simulink model "color_acquistion_test"  (R2022b)
settings: Solver=FixedStepDiscrete  StartTime=0.0  StopTime=10000.0  FixedStep=0.1  RelTol=1e-3
InitFcn:
  | mbd_s32k_consistency_checks(bdroot(gcs));
undefined symbols (not defined in the file or in its folder): LQFP
libraries: mbd_s32k1xx_ec_toolbox x5
settings Model: Creator=leona  LastModifiedBy=leona
settings DataIOCC: SaveOutput=off  SignalLogging=off  SaveTime=off
settings OptimizationCC: DefaultParameterBehavior=Inlined  EnhancedBackFolding=on  PassReuseOutputArgsAs=Individual arguments  ZeroExternalMemoryAtStartup=off  ZeroInternalMemoryAtStartup=off  OptimizeBlockOrder=speed  DifferentSizesBufferReuse=on  OptimizationCustomize=off  EfficientTunableParamExpr=on
settings DebuggingCC: InheritedTsInSrcMsg=none  SingleTaskRateTransMsg=error  ParameterTunabilityLossMsg=error  UnconnectedInputMsg=error  UnconnectedOutputMsg=error  UnconnectedLineMsg=error  UnknownTsInhSupMsg=error
settings HardwareCC: ProdBitPerPointer=32  ProdBitPerSizeT=32  ProdBitPerPtrDiffT=32  ProdLargestAtomicInteger=Long  ProdLargestAtomicFloat=Double  ProdWordSize=32  ProdHWDeviceType=ARM Compatible->ARM Cortex
settings ModelReferenceCC: ModelReferenceNumInstancesAllowed=Single
settings SFSimCC: MATLABDynamicMemAlloc=off
settings RTWCC: Description=Model Based Design Toolbox S32K1xx Code Generation Target  SystemTargetFile=mbd_s32k.tlc  MakeCommand=mbd_s32k_make_rtw COPY_MDLREF_INCLUDES=0  TemplateMakefile=mbd_s32k.tmf
settings CodeAppCC: ForceParamTrailComments=on  IgnoreCustomStorageClasses=off  OperatorAnnotations=on  SimulinkDataObjDesc=on  SFDataObjDesc=on  InsertBlockDesc=on
settings STFCustomTargetCC: TargetLangStandard=C99 (ISO)  MultiwordLength=256  CombineOutputUpdateFcns=on  ERTCustomFileBanners=on  SupportContinuousTime=off  SupportNonInlinedSFcns=off  RemoveResetFunc=on  MATLABClassNameForMDSCustomization=Simulink.SoftwareTarget.ERTCustomization  SystemTargetFile=mbd_s32k.tlc
settings ERTTargetCC: TargetLangStandard=C99 (ISO)  ParMdlRefBuildCompliant=off  CompOptLevelCompliant=off  ConcurrentExecutionCompliant=off  ModelStepFunctionPrototypeControlCompliant=off  CPPClassGenCompliant=off  UseToolchainInfoCompliant=off  ExtMode=on  InlinedParameterPlacement=NonHierarchical  ERTSrcFileBannerTemplate=mbd_ert_code_template.cgt  ERTHdrFileBannerTemplate=mbd_ert_code_template.cgt  ERTDataSrcFileTemplate=mbd_ert_code_template.cgt  ERTDataHdrFileTemplate=mbd_ert_code_template.cgt  ERTCustomFileTemplate=example_file_process.tlc

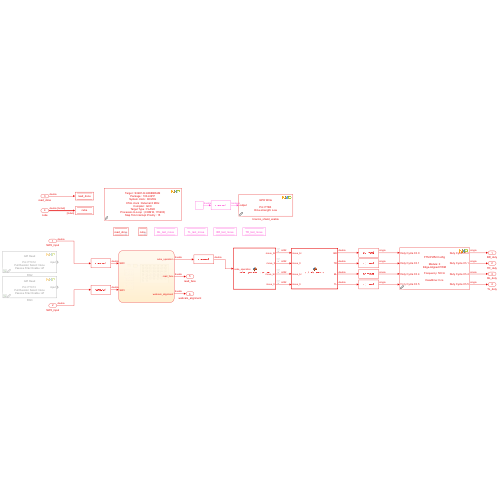
[thumbnail: Simulink's stored preview of the top-level diagram]
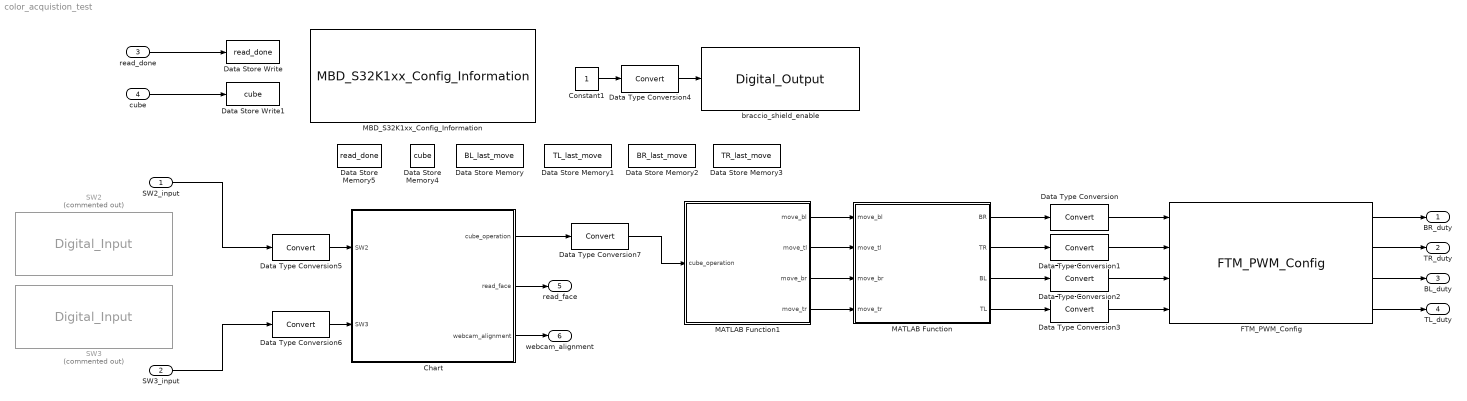
== system color_acquistion_test ==
  SW2_input : Inport
  SW3_input : Inport  Port=2
  read_done : Inport  Port=3
  cube : Inport  Port=4
  Chart : Stateflow chart  TreatAsAtomicUnit=on
  Constant1 : Constant
  Data Store Memory : DataStoreMemory  DataStoreName=BL_last_move  WriteAfterWriteMsg=warning  ShowAdditionalParam=off
  Data Store Memory1 : DataStoreMemory  DataStoreName=TL_last_move  WriteAfterWriteMsg=warning  ShowAdditionalParam=off
  Data Store Memory2 : DataStoreMemory  DataStoreName=BR_last_move  WriteAfterWriteMsg=warning  ShowAdditionalParam=off
  Data Store Memory3 : DataStoreMemory  DataStoreName=TR_last_move  WriteAfterWriteMsg=warning  ShowAdditionalParam=off
  Data Store Memory4 : DataStoreMemory  DataStoreName=cube  WriteAfterWriteMsg=warning  InitialValue=zeros(3, 3, 6)  VectorParams1D=off  ShowAdditionalParam=off  OutDataTypeStr=double
  Data Store Memory5 : DataStoreMemory  DataStoreName=read_done  WriteAfterWriteMsg=warning  ShowAdditionalParam=off  OutDataTypeStr=double
  Data Store Write : DataStoreWrite  DataStoreName=read_done  IndexOptions=Index vector (dialog)  Indices=1  OutputSizes=1
  Data Store Write1 : DataStoreWrite  DataStoreName=cube  IndexOptions=Index vector (dialog)  Indices=1  OutputSizes=1
  Data Type Conversion{,1..7} (8 alike) : DataTypeConversion  SaturateOnIntegerOverflow=off  RndMeth=Floor
  FTM_PWM_Config : mbd_s32k1xx_ec_toolbox/Motor Control Blocks/FTM Blocks/FTM_PWM_Config  ftmModule=0  ftmMode=Edge-Aligned PWM  ftmSourceClock=80 MHz  swcontrol_enable=off  chan0En=on  chan0Type=Independent  chan2En=off  chan2Type=Independent  chan4En=on  chan4Type=Independent  chan6En=off  chan6Type=Independent  ftmPwmUnits=Hz  outFrequency=50  ftmPeriod=25000  ftmPrescaler=Divide by 64  deadtimeUnits=Nanoseconds  deadtimeNs=0  deadtimeTicks=0  deadtimePrescaler=Divide by 1  dutyCycleCh0=0.03  dutyCycleCh1=0.125  dutyCycleCh2=0.025  dutyCycleCh3=0.025  dutyCycleCh4=0.025  dutyCycleCh5=0.025  dutyCycleCh6=0.25  dutyCycleCh7=0.25  dutyCycleSim=on  startAfterInit=on  showAdvOpt=on  pinFtmCh0=PTD15: [FTM0_CH0 | FTM Channel]  pinFtmCh1=PTD16: [FTM0_CH1 | FTM Channel]  pinPolCh0=Active High  pinPolCh1=Active High  outputComplem0=Main duplicated  outputLevel0=Low  outputLevel1=Low  pinFtmCh2=PTB14: [FTM0_CH2 | FTM Channel]  pinFtmCh3=PTC3: [FTM0_CH3 | FTM Channel]  pinPolCh2=Active High  pinPolCh3=Active High  outputComplem2=Main duplicated  outputLevel2=Low  outputLevel3=Low  pinFtmCh4=PTB4: [FTM0_CH4 | FTM Channel]  pinFtmCh5=PTB5: [FTM0_CH5 | FTM Channel]  pinPolCh4=Active High  pinPolCh5=Active High  outputComplem4=Main duplicated  outputLevel4=Low  outputLevel5=Low  pinFtmCh6=PTE8: [FTM0_CH6 | FTM Channel]  pinFtmCh7=None  pinPolCh6=Active High  pinPolCh7=Active High  outputComplem6=Main duplicated  outputLevel6=Low  outputLevel7=Low  initTrigger=off  chTrigger0=off  chTrigger1=off  chTrigger2=off  chTrigger3=off  chTrigger4=off  chTrigger5=off  chTrigger6=off  chTrigger7=off  mcuTargetUpdate=on  pwmSyncTrg=Software trigger  pwmSyncHwRouting=TRGMUX_FTM7  pwmSyncTrg0=off  pwmSyncTrg1=off  pwmSyncTrg2=off  pwmSyncAutoClear=on  pwmSyncMinLoad=on  pwmSyncMaxLoad=on  pwmSyncInvert=System Clock  pwmSyncOutControl=System Clock  pwmSyncOutMask=System Clock  pwmSyncCounterInitial=System Clock  pwmSyncPoints=Update now  reloadEnable=off  reloadPriority=15  reloadHalfCycle=off  reloadHCR=0  reloadFrequency=0  chnMatch0=off  chnMatch1=off  chnMatch2=off  chnMatch3=off  chnMatch4=off  chnMatch5=off  chnMatch6=off  chnMatch7=off  pwmFaultProtection=off  pwmFaultInterrupt=off  pwmFaultClearing=Fault control disabled  pwmFaultPinState=Safe Value  pwmFaultFilterValue=0  pwmFaultPriority=15  fault_disen_0=off  fault_filter_0=off  fault_polarity_0=Active High  fault_disen_1=off  fault_filter_1=off  fault_polarity_1=Active high  fault_disen_2=off  fault_filter_2=off  fault_polarity_2=Active high  fault_disen_3=off  fault_filter_3=off  fault_polarity_3=Active high  fault_pin_0=None  fault_pin_1=None  fault_pin_2=None  fault_pin_3=None
  MATLAB Function : MATLAB Function  TreatAsAtomicUnit=on
  MATLAB Function1 : MATLAB Function  TreatAsAtomicUnit=on
  MBD_S32K1xx_Config_Information : mbd_s32k1xx_ec_toolbox/MBD_S32K1xx_Config_Information  mbdt_ver=0  disp_str=|  config_params=[]  mcu_target_name=S32K144  mcu_target_package=100-LQFP  mcu_target_sram_size=48KB  mcu_system_clock_freq=80  mcu_xtal_freq=External 8  mcu_steptick_timer=LPIT Channel 0  mcu_steptick_prio=15  ds_import_enable=on  target_compiler=GCC  target_memory=FLASH  gcc_target_compile_opts=-mthumb -mfloat-abi=hard -mfpu=fpv4-sp-d16 -O1 -g -gstrict-dwarf  gcc_target_assemble_opts=-mthumb -mfloat-abi=hard -mfpu=fpv4-sp-d16 -g  gcc_target_link_opts=-mthumb -mfloat-abi=hard -mfpu=fpv4-sp-d16  gcc_target_default_lcf=on  gcc_target_user_lcf=S32K144_48_flash.ld  ghs_target_compile_opts=-cpu=cortexm4f -thumb -fpu=vfpv4_d16 -fsingle -Ogeneral -Wundef -Wimplicit-int -Wshadow -Wtrigraphs --no_commons --gnu_asm -gnu99 -gdwarf-2 -G  ghs_target_assemble_opts=-cpu=cortexm4f -fpu=vfpv4_d16  ghs_target_link_opts=-cpu=cortexm4f -thumb -fpu=vfpv4_d16  ghs_target_default_lcf=on  ghs_target_user_lcf=S32K144_48_flash.ld  iar_target_compile_opts=--cpu=Cortex-M4F --thumb --fpu=VFPv4_sp -Ol -e --debug --dlib_config normal  iar_target_assemble_opts=--cpu Cortex-M4F --thumb --fpu VFPv4_sp  iar_target_link_opts=--no_exceptions --vfe --inline  iar_target_default_lcf=on  iar_target_user_lcf=S32K144_48_flash.icf  pil_download_enable=on  rbl_download_enable=on  rbl_start_delay=5000  rbl_download_interface=OpenSDA  rbl_restart_request=off  rbl_com_port=Custom  rbl_com_port_custom=COM18  pil_download_rate=115200  pil_download_rate_custom=115200  pil_opensda_drive=Custom  pil_opensda_drive_custom=D  jtag_interface=OpenSDA Embedded Debug  jlink_default_path=on  jlink_user_path=C:\Program Files\SEGGER\JLink\  pil_uart_instance=1  pil_uart_rx=PTC6: [LPUART1_RX | Receive]  pil_uart_tx=PTC7: [LPUART1_TX | Transmit]  FTM_PWM_PcrCheckEnDis=on  FTM_Input_Edge_Inputs_PcrCheckEnDis=on  FTM_Dual_Edge_Inputs_PcrCheckEnDis=on  FTM_Quadrature_Inputs_PcrCheckEnDis=on  FTM_Hall_Sensor_Inputs_PcrCheckEnDis=on  LPTMR_PcrCheckEnDis=on  PIT_PcrCheckEnDis=on  RTC_PcrCheckEnDis=on  FlexCAN_PcrCheckEnDis=on  LIN_PcrCheckEnDis=on  FlexIO_PcrCheckEnDis=on  LPI2C_PcrCheckEnDis=on  LPSPI_PcrCheckEnDis=on  LPUART_PcrCheckEnDis=on  CMP_PcrCheckEnDis=on  GPIO_OutputPcrCheckEnDis=on  GPIO_InputPcrCheckEnDis=on  SBC_PcrCheckEnDis=on  BMS_PcrCheckEnDis=on  AMMCLIB_PcrCheckEnDis=on  FM_PcrCheckEnDis=on  Profile_PcrCheckEnDis=on  ConfigParams_PcrCheckEnDis=on  ModelRef_PcrCheckEnDis=on  PDB0_PcrCheckEnDis=on  CSEc_PcrCheckEnDis=on  eDMA_PcrCheckEnDis=on  FLASH_PcrCheckEnDis=on  ADC_PcrCheckEnDis=on  WDOG_PcrCheckEnDis=on
      | Target : S32K144-64KB_SRAM
      | Package : 100-pin
      | System clock : 80 MHz
      | XTAL clock : External 8 MHz
      | Compiler : IAR
      | Target Type : FLASH
      | Download Code after build : off
      | Step Tick Interrupt Priority : 15
  SW2 : mbd_s32k1xx_ec_toolbox/GPIO Blocks/Digital_Input  Commented=on  gpio_pin=PTC12: [PTC12 | Port C I/O]  pull_resistor=None  passive_filter=off
  SW3 : mbd_s32k1xx_ec_toolbox/GPIO Blocks/Digital_Input  Commented=on  gpio_pin=PTC13: [PTC13 | Port C I/O]  pull_resistor=None  passive_filter=off
  braccio_shield_enable : mbd_s32k1xx_ec_toolbox/GPIO Blocks/Digital_Output  gpio_pin=PTB3: [PTB3 | Port B I/O]  init_val=Low  drive_strength=Low
  BR_duty : Outport
  TR_duty : Outport  Port=2
  BL_duty : Outport  Port=3
  TL_duty : Outport  Port=4
  read_face : Outport  Port=5
  webcam_alignment : Outport  Port=6
  wires:
  Data Type Conversion2/1 -> FTM_PWM_Config/3
  MATLAB Function1/3(move_br) -> MATLAB Function/3(move_br)
  FTM_PWM_Config/1 -> BR_duty/1
  MATLAB Function/4(TL) -> Data Type Conversion3/1
  FTM_PWM_Config/2 -> TR_duty/1
  Data Type Conversion5/1 -> Chart/1(SW2)
  Data Type Conversion4/1 -> braccio_shield_enable/1
  MATLAB Function/3(BL) -> Data Type Conversion2/1
  Chart/1(cube_operation) -> Data Type Conversion7/1
  Constant1/1 -> Data Type Conversion4/1
  MATLAB Function/1(BR) -> Data Type Conversion/1
  MATLAB Function1/1(move_bl) -> MATLAB Function/1(move_bl)
  FTM_PWM_Config/4 -> TL_duty/1
  Data Type Conversion7/1 -> MATLAB Function1/1(cube_operation)
  FTM_PWM_Config/3 -> BL_duty/1
  Data Type Conversion3/1 -> FTM_PWM_Config/4
  MATLAB Function/2(TR) -> Data Type Conversion1/1
  Data Type Conversion6/1 -> Chart/2(SW3)
  Data Type Conversion1/1 -> FTM_PWM_Config/2
  MATLAB Function1/4(move_tr) -> MATLAB Function/4(move_tr)
  Data Type Conversion/1 -> FTM_PWM_Config/1
  MATLAB Function1/2(move_tl) -> MATLAB Function/2(move_tl)
  SW2_input/1 -> Data Type Conversion5/1
  SW3_input/1 -> Data Type Conversion6/1
  Chart/2(read_face) -> read_face/1
  Chart/3(webcam_alignment) -> webcam_alignment/1
  read_done/1 -> Data Store Write/1
  cube/1 -> Data Store Write1/1

== matlab function color_acquistion_test/MATLAB Function1 ==
  data: cube_operation input; move_bl output; move_tl output; move_br output; move_tr output
function [move_bl, move_tl, move_br, move_tr] = cube_operation_decoder(cube_operation)
% This function takes as input the code for a cube operation and converts
% it as positions of the 4 servo motors. The operations must be a 4 digit
% unsigned integer, encoded as follows:
%   - first digit [0, 1]: open/close left grip;
%   - second digit [0, 1]: open/close right grip;
%   - third digit [0, 1, 2]: set left arm to 90/0/180 degrees
%   - fourth digit [0, 1, 2]: set right arm to 90/0/180 degress

x1 = int32(mod(cube_operation/1000, 10));
x2 = int32(mod(cube_operation/100, 10));
x3 = int32(mod(cube_operation/10, 10));
x4 = int32(mod(cube_operation, 10));

move_tl = x1;
move_tr = x2;
move_bl = x3;
move_br = x4;

== matlab function color_acquistion_test/MATLAB Function ==
  data: BR output; TR output; move_bl input; BL output; move_tl input; move_br input; move_tr input; TL output
function [BR, TR, BL, TL] = actuate_servos(move_bl, move_tl, move_br, move_tr)
% This function takes as input as specific number associated to a movement
% of the 4 servo motors (BL = Bottom Left, TL = Top Left, BR = Bottom Right,
% TR = Top Right) and it gives as output the 4 relative duty cycles needed to
% obtain that movement. 

min_duty = 0.025;
max_duty = 0.125;

duty_0_deg = min_duty;
duty_grip_open = min_duty + (max_duty-min_duty)/3;
duty_grip_closed = min_duty + (max_duty-min_duty)/15; 
duty_90_deg = min_duty + (max_duty-min_duty)/2;
duty_180_deg = max_duty;

switch (move_tl)
    case 0                  % Open left grip
        TL = duty_grip_open;
    case 1                  % Close left grip
        TL = duty_grip_closed;
    otherwise               % Open left grip
        TL = duty_grip_open;
end

switch (move_tr)
    case 0                  % Open right grip
        TR = duty_grip_open;
    case 1                  % Close right grip
        TR = duty_grip_closed;
    otherwise               % Open right grip
        TR = duty_grip_open;
end

switch (move_bl)
    case 0                  % Left arm straight
        BL = duty_90_deg;
    case 1                  % Left arm at 90° clockwise
        BL = duty_0_deg;
    case 2                 % Left arm at 90° counter-clockwise
        BL = duty_180_deg;
    otherwise
        BL = duty_90_deg;
end

switch (move_br)
    case 0                  % Right arm straight
        BR = duty_90_deg;
    case 1                  % Right arm at 90° clockwise
        BR = duty_0_deg;
    case 2                 % Right arm at 90° counter-clockwise
        BR = duty_180_deg;
    otherwise
        BR = duty_90_deg;
end

% Update current position of the motors
BL_last_move = move_bl;
TL_last_move = move_tl;
BR_last_move = move_br;
TR_last_move = move_tr;

== stateflow chart color_acquistion_test/Chart ==
  state read_cube
    en:
    webcam_alignment = 0;
    % Clear cube colors
    cube = zeros(3, 3, 6);
    %read red
    %LTm
    %read blue
    %LTm
    %read orange
    %LTm
    %read green
    %RTm
    %LTm
    %read white
    %RTmm
    %LTmm
    %read yellow
    %RTm
    %LTm
    %RTp
    state read_red
      en:
    state fase1e
      en:
      cube_operation=1000
    state fase2e
      en:
      cube_operation=1010
    state fase3e
      en:
      cube_operation=1110
    state fase4e
      en:
      cube_operation=0110
    state fase5e
      en:
      cube_operation=0100
    state fase6er
      en:
      cube_operation=1100
    state fase12e
      en:
      cube_operation=1100
    state fase11e
      en:
      cube_operation=0100
    state fase10e
      en:
      cube_operation=0110
    state fase9e
      en:
      cube_operation=1110
    state fase8e
      en:
      cube_operation=1010
    state fase7e
      en:
      cube_operation=1000
    state read_blue
      en:
    state read_orange
      en:
    state fase13e
      en:
      cube_operation=1000
    state fase14e
      en:
      cube_operation=1010
    state fase15e
      en:
      cube_operation=1110
    state fase16e
      en:
      cube_operation=0110
    state fase17e
      en:
      cube_operation=0100
    state fase18e
      en:
      cube_operation=1100
    state fase24e
      en:
      cube_operation=1100
    state fase23e
      en:
      cube_operation=1000
    state fase22e
      en:
      cube_operation=1001
    state fase21e
      en:
      cube_operation=1101
    state fase20e
      en:
      cube_operation=0101
    state fase19e
      en:
      cube_operation=0100
    state read_green
      en:
    state fase27e
      en:
      cube_operation=1110
    state fase25e
      en:
      cube_operation=1000
    state fase26e
      en:
      cube_operation=1010
    state fase28e
      en:
      cube_operation=0110
    state fase29e
      en:
      cube_operation=0100
    state fase30e
      en:
      cube_operation=1100
    state read_white
      en:
    state fase35e
      en:
      cube_operation=1000
    state fase37e
      en:
      cube_operation=0100
    state fase36e
      en:
      cube_operation=1100
    state fase34e
      en:
      cube_operation=1001
    state fase33e
      en:
      cube_operation=1101
    state fase32e
      en:
      cube_operation=0101
    state fase31e
      en:
      cube_operation=0100
    state fase38e
      en:
      cube_operation=0101
    state fase39e
      en:
      cube_operation=1101
    state fase40e
      en:
      cube_operation=1001
    state fase41e
      en:
      cube_operation=1000
    state fase42e
      en:
      cube_operation=1100
    state fase43e
      en:
      cube_operation=1000
    state fase44e
      en:
      cube_operation=1010
    state fase51w
      en:
      cube_operation=1110
    state fase50e
      en:
      cube_operation=1010
    state fase49e
      en:
      cube_operation=1000
    state fase48e
      en:
      cube_operation=1100
    state fase47e
      en:
      cube_operation=0100
    state fase46e
      en:
      cube_operation=0110
    state fase45e
      en:
      cube_operation=1110
    state read_yellow
      en:
    state fase55e
      en:
      cube_operation=0100
    state fase56e
      en:
      cube_operation=0101
    state fase57e
      en:
      cube_operation=1101
    state fase52e
      en:
      cube_operation=0110
    state fase54e
      en:
      cube_operation=1100
    state fase53e
      en:
      cube_operation=0100
    state fase58e
      en:
      cube_operation=1001
    state fase63e
      en:
      cube_operation=1110
    state fase64e
      en:
      cube_operation=0110
    state fase62e
      en:
      cube_operation=1010
    state fase61e
      en:
      cube_operation=1000
    state fase60e
      en:
      cube_operation=1100
    state fase59e
      en:
      cube_operation=1000
    state fase65e
      en:
      cube_operation=0100
    state fase66e
      en:
      cube_operation=1100
    (default) -> read_red
    read_red -> fase1e
    fase1e -> fase2e : [after(delay_ms, msec)]
    fase2e -> fase3e : [after(delay_ms, msec)]
    fase3e -> fase4e : [after(delay_ms, msec)]
    fase4e -> fase5e : [after(delay_ms, msec)]
    fase5e -> fase6er : [after(delay_ms, msec)]
    fase6er -> read_blue : [after(delay_ms, msec)]
    fase11e -> fase12e : [after(delay_ms, msec)]
    fase10e -> fase11e : [after(delay_ms, msec)]
    fase9e -> fase10e : [after(delay_ms, msec)]
    fase8e -> fase9e : [after(delay_ms, msec)]
    fase7e -> fase8e : [after(delay_ms, msec)]
    read_blue -> fase7e : [after(delay_ms, msec)]
    fase12e -> read_orange : [after(delay_ms, msec)]
    read_orange -> fase13e : [after(delay_ms, msec)]
    fase13e -> fase14e : [after(delay_ms, msec)]
    fase14e -> fase15e : [after(delay_ms, msec)]
    fase15e -> fase16e : [after(delay_ms, msec)]
    fase16e -> fase17e : [after(delay_ms, msec)]
    fase17e -> fase18e : [after(delay_ms, msec)]
    fase18e -> read_green : [after(delay_ms, msec)]
    fase23e -> fase24e : [after(delay_ms, msec)]
    fase22e -> fase23e : [after(delay_ms, msec)]
    fase21e -> fase22e : [after(delay_ms, msec)]
    fase20e -> fase21e : [after(delay_ms, msec)]
    fase19e -> fase20e : [after(delay_ms, msec)]
    read_green -> fase19e : [after(delay_ms, msec)]
    fase24e -> fase25e : [after(delay_ms, msec)]
    fase26e -> fase27e : [after(delay_ms, msec)]
    fase27e -> fase28e : [after(delay_ms, msec)]
    fase25e -> fase26e : [after(delay_ms, msec)]
    fase28e -> fase29e : [after(delay_ms, msec)]
    fase29e -> fase30e : [after(delay_ms, msec)]
    fase30e -> read_white : [after(delay_ms, msec)]
    read_white -> fase31e : [after(delay_ms, msec)]
    fase35e -> fase36e : [after(delay_ms, msec)]
    fase34e -> fase35e : [[after(delay_ms, msec)]]
    fase36e -> fase37e : [after(delay_ms, msec)]
    fase33e -> fase34e : [after(delay_ms, msec)]
    fase32e -> fase33e : [after(delay_ms, msec)]
    fase31e -> fase32e : [after(delay_ms, msec)]
    fase37e -> fase38e : [after(delay_ms, msec)]
    fase39e -> fase40e : [after(delay_ms, msec)]
    fase38e -> fase39e : [after(delay_ms, msec)]
    fase40e -> fase41e : [after(delay_ms, msec)]
    fase41e -> fase42e : [after(delay_ms, msec)]
    fase42e -> fase43e : [after(delay_ms, msec)]
    fase43e -> fase44e : [after(delay_ms, msec)]
    fase44e -> fase45e : [after(delay_ms, msec)]
    fase49e -> fase50e : [after(delay_ms, msec)]
    fase48e -> fase49e : [after(delay_ms, msec)]
    fase46e -> fase47e : [after(delay_ms, msec)]
    fase45e -> fase46e : [after(delay_ms, msec)]
    fase50e -> fase51w : [after(delay_ms, msec)]
    fase47e -> fase48e : [after(delay_ms, msec)]
    fase51w -> fase52e : [after(delay_ms, msec)]
    fase56e -> fase57e : [after(delay_ms, msec)]
    fase54e -> read_yellow : [after(delay_ms, msec)]
    fase55e -> fase56e : [after(delay_ms, msec)]
    read_yellow -> fase55e : [after(delay_ms, msec)]
    fase52e -> fase53e : [after(delay_ms, msec)]
    fase53e -> fase54e : [after(delay_ms, msec)]
    fase57e -> fase58e : [after(delay_ms, msec)]
    fase62e -> fase63e : [after(delay_ms, msec)]
    fase61e -> fase62e : [after(delay_ms, msec)]
    fase60e -> fase61e : [after(delay_ms, msec)]
    fase59e -> fase60e : [after(delay_ms, msec)]
    fase63e -> fase64e : [after(delay_ms, msec)]
    fase58e -> fase59e : [after(delay_ms, msec)]
    fase64e -> fase65e : [after(delay_ms, msec)]
    fase65e -> fase66e : [after(delay_ms, msec)]
  state webcam_alignment
    en:
    SW2_status = SW2;
    SW3_status = SW3;
    cube_operation=1100;
    webcam_alignment = 1;
    du:
    SW2_status=SW2;
    SW3_status=SW3;
  state wait_cube
    en:
    SW2_status = SW2;
    cube_operation=0100;
    du:
    SW2_status=SW2;
  state Li [commented out]
    en:
    %LTpp
    %RMm
    state fase1 [commented out]
      en:
      %cube_operation=0100;
      cube_operation=0110;
    state fase2 [commented out]
      en:
      cube_operation=1110;
    state fase3 [commented out]
      en:
      %cube_operation=1010;
      cube_operation=1020;
    state fase5 [commented out]
      en:
      %cube_operation=0120;
      cube_operation=0100;
    state fase4 [commented out]
      en:
      cube_operation=1120;
    state fase6 [commented out]
      en:
      cube_operation=1100
    state fase9 [commented out]
      en:
      cube_operation=1100;
    state fase8 [commented out]
      en:
      %cube_operation=1001;
      cube_operation=1000;
    state fase7 %RMm [commented out]
      en:
      cube_operation=1101;
    (default) -> Li.fase1 [commented out]
    Li.fase1 -> Li.fase2 [commented out] : [after(500,msec)]
    Li.fase2 -> Li.fase3 [commented out] : [after(500,msec)]
    Li.fase3 -> Li.fase4 [commented out] : [after(500,msec)]
    Li.fase4 -> Li.fase5 [commented out] : [after(500,msec)]
    Li.fase5 -> Li.fase6 [commented out] : [after(500,msec)]
    Li.fase6 -> fase7 %RMm [commented out] : [after(500,msec)]
    Li.fase8 -> Li.fase9 [commented out] : [after(500,msec)]
    fase7 %RMm -> Li.fase8 [commented out] : [after(500,msec)]
  state L [commented out]
    en:
    %LTpp
    %RMp
    state fase1 [commented out]
      en:
      %cube_operation=0100;
      cube_operation=0110;
    state fase2 [commented out]
      en:
      cube_operation=1110;
    state fase3 [commented out]
      en:
      %cube_operation=1010;
      cube_operation=1020;
    state fase5 [commented out]
      en:
      %cube_operation=0120;
      cube_operation=0100;
    state fase4 [commented out]
      en:
      cube_operation=1120;
    state fase6 [commented out]
      en:
      cube_operation=1100
    state fase9 [commented out]
      en:
      cube_operation=1100;
    state fase8 [commented out]
      en:
      cube_operation=1101;
    state fase7 %RMp [commented out]
      en:
      %cube_operation=1000;
      cube_operation=1001;
    (default) -> L.fase1 [commented out]
    L.fase1 -> L.fase2 [commented out] : [after(500,msec)]
    L.fase2 -> L.fase3 [commented out] : [after(500,msec)]
    L.fase3 -> L.fase4 [commented out] : [after(500,msec)]
    L.fase4 -> L.fase5 [commented out] : [after(500,msec)]
    L.fase5 -> L.fase6 [commented out] : [after(500,msec)]
    L.fase6 -> fase7 %RMp [commented out] : [after(500,msec)]
    L.fase8 -> L.fase9 [commented out] : [after(500,msec)]
    fase7 %RMp -> L.fase8 [commented out] : [after(500,msec)]
  state L2 [commented out]
    en:
    %LTpp
    %RMpp
    state fase1 [commented out]
      en:
      %cube_operation=0100;
      cube_operation=0110;
    state fase2 [commented out]
      en:
      cube_operation=1110;
    state fase3 [commented out]
      en:
      %cube_operation=1010;
      cube_operation=1020;
    state fase5 [commented out]
      en:
      %cube_operation=0120;
      cube_operation=0100;
    state fase4 [commented out]
      en:
      cube_operation=1120;
    state fase6 [commented out]
      en:
      cube_operation=1100
    state fase9 [commented out]
      en:
      cube_operation=1102;
    state fase8 [commented out]
      en:
      cube_operation=1101;
    state fase7 %RMpp [commented out]
      en:
      %cube_operation=1000;
      cube_operation=1001;
    state fase10 [commented out]
      en:
      %cube_operation=1002;
      cube_operation=1000;
    state fase11 [commented out]
      en:
      cube_operation=1100;
    (default) -> L2.fase1 [commented out]
    L2.fase1 -> L2.fase2 [commented out] : [after(500,msec)]
    L2.fase2 -> L2.fase3 [commented out] : [after(500,msec)]
    L2.fase3 -> L2.fase4 [commented out] : [after(500,msec)]
    L2.fase4 -> L2.fase5 [commented out] : [after(500,msec)]
    L2.fase5 -> L2.fase6 [commented out] : [after(500,msec)]
    L2.fase6 -> fase7 %RMpp [commented out] : [after(500,msec)]
    L2.fase8 -> L2.fase9 [commented out] : [after(500,msec)]
    fase7 %RMpp -> L2.fase8 [commented out] : [after(500,msec)]
    L2.fase9 -> fase10 [commented out] : [after(500,msec)]
    fase10 -> fase11 [commented out] : [after(500,msec)]
  (default) -> wait_cube
  wait_cube -> webcam_alignment : [SW2==1 && SW2_status==0]
  webcam_alignment -> read_cube [order 2] : [SW3==1 && SW3_status==0]
  webcam_alignment -> wait_cube [order 1] : [SW2==1 && SW2_status==0]
  data: SW2 input; cube_operation output; SW3 input; SW3_status local =0; SW2_status local double =0; delay_ms constant double =200; cube data_store_memory; read_face output =0; webcam_alignment output =0; read_done data_store_memory
